simulink model "asbCubeSatACS"  (R2025b)
settings: Solver=FixedStepDiscrete  StartTime=0.0  StopTime=1000  FixedStep=CubeSatTimeStep  RelTol=1e-3  EnableMultiTasking=on
libraries: sharedtransform x2, aerolibsatdyn x1, aerolibutil x1
settings Model: DataDictionary=asbCubeSatModelData.sldd  ExtModeAutoUpdateStatusClock=off  Creator=The MathWorks, Inc.  LastModifiedBy=alokahn
settings SolverCC: AlgebraicLoopSolver=TrustRegion  MaxZcPerStep=1.0
settings DataIOCC: LimitDataPoints=on  SaveFormat=Array  SaveOutput=off  SignalLogging=off  DSMLogging=off  SaveTime=off  ReturnWorkspaceOutputs=off
settings OptimizationCC: DefaultParameterBehavior=Inlined  OptimizeBlockIOStorage=off  BufferReuse=off  GlobalBufferReuse=off  ExpressionFolding=off  ExpressionDepthLimit=2147483647.0  LocalBlockOutputs=off  InitFltsAndDblsToZero=on  LifeSpan=inf  OptimizeDataStoreBuffers=off  BusAssignmentInplaceUpdate=off
settings DebuggingCC: ArtificialAlgebraicLoopMsg=none  SolverPrmCheckMsg=warning  FcnCallInpInsideContextMsg=warning  UnconnectedInputMsg=warning  UnconnectedOutputMsg=warning  UnconnectedLineMsg=warning  StateNameClashWarn=warning  PregeneratedLibrarySubsystemCodeDiagnostic=none  SFUnexpectedBacktrackingDiag=warning  SFNoUnconditionalDefaultTransitionDiag=warning  SFExecutionAtInitializationDiag=none  ArithmeticOperatorsInVariantConditions=warning
settings HardwareCC: ProdBitPerPointer=32.0  ProdBitPerSizeT=32.0  ProdBitPerPtrDiffT=32.0  ProdLargestAtomicFloat=None  ProdIntDivRoundTo=Undefined  ProdEndianess=Unspecified  ProdWordSize=32.0  ProdHWDeviceType=32-bit Generic
settings ModelReferenceCC: EnableRefExpFcnMdlSchedulingChecks=on  PropagateSignalLabelsOutOfModel=off
settings SFSimCC: SimUseLocalCustomCode=off
settings RTWCC: RTWUseLocalCustomCode=off  GPUComputeCapability=3.5  DLArmComputeVersion=19.05
settings CodeAppCC: StateflowObjectComments=on
settings GRTTargetCC: TargetFcnLib=ansi_tfl_tmw.mat  TargetLangStandard=C89/C90 (ANSI)  CombineOutputUpdateFcns=off  GRTInterface=on
settings ConfigComp: CovMetricSettings=dw  CovSaveCumulativeToWorkspaceVar=on  CovSaveSingleToWorkspaceVar=on  CovExternalEMLEnable=off

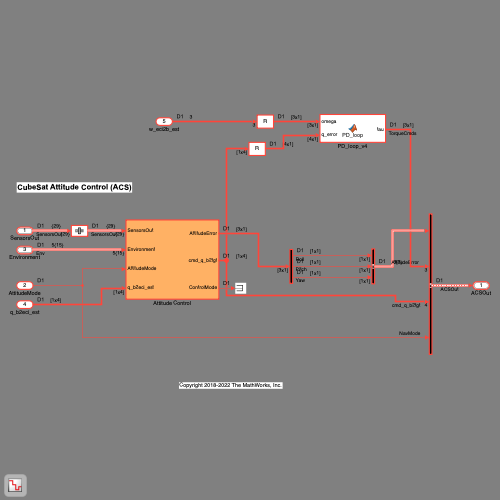
[thumbnail: Simulink's stored preview of the top-level diagram]
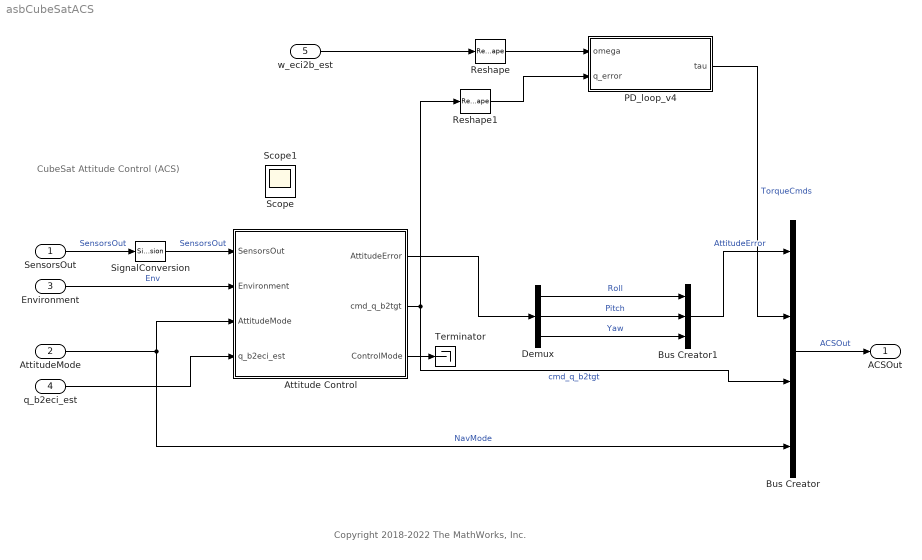
== system asbCubeSatACS ==
  note: Copyright 2018-2022 The MathWorks, Inc.
  note: CubeSat Attitude Control (ACS)
  SensorsOut : Inport  OutDataTypeStr=Bus: StatesOutBus
  AttitudeMode : Inport  Port=2  OutDataTypeStr=double  PortDimensions=1
  Environment : Inport  Port=3  OutDataTypeStr=Bus: EnvBus  PortDimensions=1
  q_b2eci_est : Inport  Port=4  PortDimensions=[1,4]  SampleTime=1
  w_eci2b_est : Inport  Port=5  SampleTime=1
  Attitude Control : Subsystem
  Bus Creator : BusCreator  Inputs=4  OutDataTypeStr=Bus: ACSOutBus  NonVirtualBus=on
  Bus Creator1 : BusCreator  Inputs=3  OutDataTypeStr=Bus: AttitudeErrorBus
  Demux : Demux  Outputs=3
  PD_loop_v4 : MATLAB Function  TreatAsAtomicUnit=on  SystemSampleTime=1
  Reshape : Reshape  OutputDimensionality=Customize  OutputDimensions=[3,1]
  Reshape1 : Reshape  OutputDimensionality=Customize  OutputDimensions=[4, 1]
  SignalConversion : SignalConversion  ConversionOutput=Virtual bus  OverrideOpt=off
  Terminator : Terminator
  ACSOut : Outport  OutDataTypeStr=Bus: ACSOutBus  PortDimensions=1  VectorParamsAs1DForOutWhenUnconnected=off  BusOutputAsStruct=on
  Scope : Scope
  Scope1 : Scope
      settings: ActiveDisplayYMinimum=-0.13646382044925889  ActiveDisplayYMaximum=3.23106670458966
  wires:
  Demux/1 -> Bus Creator1/1  "Roll"
  AttitudeMode/1 -> Bus Creator/4, Attitude Control/3("AttitudeMode ")  "NavMode"
  Demux/2 -> Bus Creator1/2  "Pitch"
  SensorsOut/1 -> SignalConversion/1  "SensorsOut"
  Bus Creator1/1 -> Bus Creator/1  "AttitudeError"
  Demux/3 -> Bus Creator1/3  "Yaw"
  Bus Creator/1 -> ACSOut/1  "ACSOut"
  Attitude Control/3(" ControlMode") -> Terminator/1
  Environment/1 -> Attitude Control/2(Environment)  "Env"
  Attitude Control/2(cmd_q_b2tgt) -> Reshape1/1, Bus Creator/3  "cmd_q_b2tgt"
  SignalConversion/1 -> Attitude Control/1("SensorsOut ")  "SensorsOut"
  Reshape/1 -> PD_loop_v4/1(omega)
  Attitude Control/1(AttitudeError) -> Demux/1
  PD_loop_v4/1(tau) -> Bus Creator/2  "TorqueCmds"
  Reshape1/1 -> PD_loop_v4/2(q_error)
  q_b2eci_est/1 -> Attitude Control/4(q_b2eci_est)
  w_eci2b_est/1 -> Reshape/1

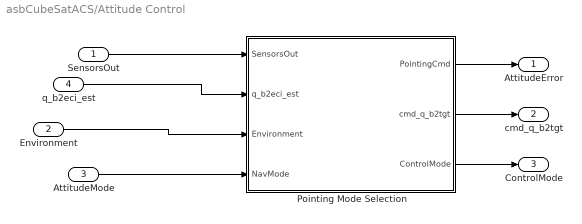
== system asbCubeSatACS/Attitude Control ==
  "SensorsOut " : Inport  OutDataTypeStr=Bus: StatesOutBus
  Environment : Inport  Port=2
  "AttitudeMode " : Inport  Port=3
  q_b2eci_est : Inport  Port=4  PortDimensions=[1,4]
  Pointing Mode Selection : Stateflow chart  RequirementInfo="{}  %GIDa_a065c7c8_537d_4123_b3cc_6e7e7008a32c"  TreatAsAtomicUnit=on
  AttitudeError : Outport  VectorParamsAs1DForOutWhenUnconnected=off
  cmd_q_b2tgt : Outport  Port=2  VectorParamsAs1DForOutWhenUnconnected=off
  " ControlMode" : Outport  Port=3  VectorParamsAs1DForOutWhenUnconnected=off
  wires:
  "SensorsOut "/1 -> Pointing Mode Selection/1(SensorsOut)
  Pointing Mode Selection/3(ControlMode) -> " ControlMode"/1
  "AttitudeMode "/1 -> Pointing Mode Selection/4(NavMode)
  Environment/1 -> Pointing Mode Selection/3(Environment)
  Pointing Mode Selection/1(PointingCmd) -> AttitudeError/1
  Pointing Mode Selection/2(cmd_q_b2tgt) -> cmd_q_b2tgt/1
  q_b2eci_est/1 -> Pointing Mode Selection/2(q_b2eci_est)

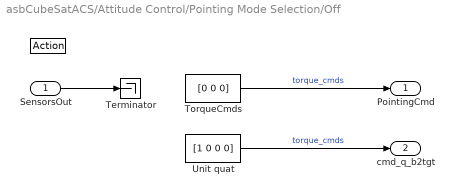
== system asbCubeSatACS/Attitude Control/Pointing Mode Selection/Off ==
  SensorsOut : Inport  OutDataTypeStr=Bus: StatesOutBus
  " " : ActionPort
      settings: CopyFcn=Stateflow.SLINSF.SimulinkMan.removeBlockPreDeleteFcn  PreDeleteFcn=Stateflow.SLINSF.SimulinkMan.unsafePredeleteFcn
  Terminator : Terminator
  TorqueCmds : Constant  Value=[0 0 0]
  Unit quat : Constant  Value=[1 0 0 0]
  PointingCmd : Outport  RequirementInfo="{}  %GIDa_4dc055f9_6cac_42e1_8ddb_4145586b89f5"  VectorParamsAs1DForOutWhenUnconnected=off
  cmd_q_b2tgt : Outport  RequirementInfo="{}  %GIDa_ca05d0a6_a581_4c3e_b3a0_cd281b586de8"  Port=2  VectorParamsAs1DForOutWhenUnconnected=off
  wires:
  SensorsOut/1 -> Terminator/1
  TorqueCmds/1 -> PointingCmd/1  "torque_cmds"
  Unit quat/1 -> cmd_q_b2tgt/1  "torque_cmds"

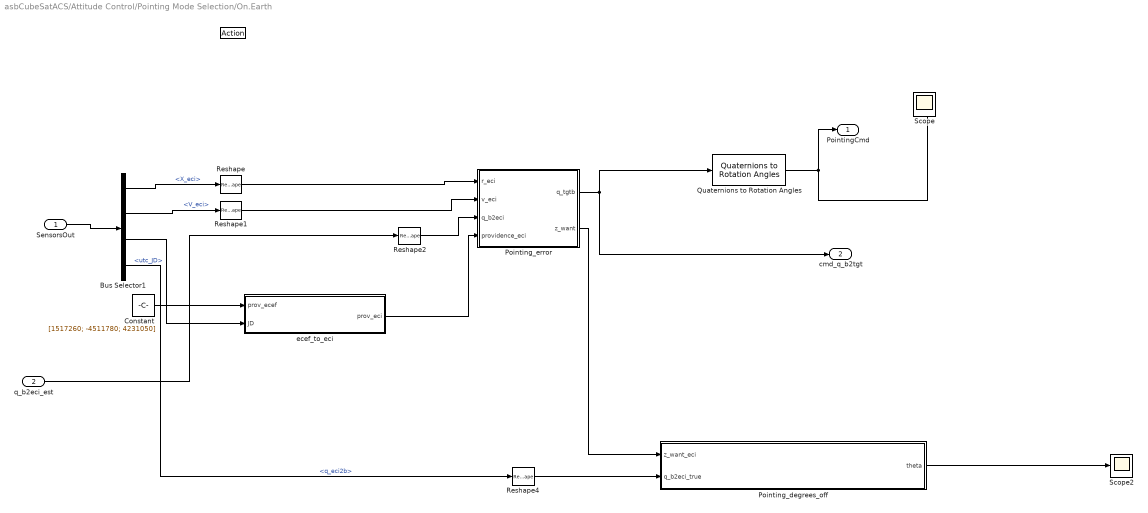
== system asbCubeSatACS/Attitude Control/Pointing Mode Selection/On.Earth ==
  SensorsOut : Inport  OutDataTypeStr=Bus: StatesOutBus
  q_b2eci_est : Inport  Port=2  PortDimensions=[1,4]
  " " : ActionPort
      settings: CopyFcn=Stateflow.SLINSF.SimulinkMan.removeBlockPreDeleteFcn  PreDeleteFcn=Stateflow.SLINSF.SimulinkMan.unsafePredeleteFcn
  Bus Selector1 : BusSelector  OutputSignals=X_eci,V_eci,utc_JD,q_eci2b
  Constant : Constant  Value=[1517260; -4511780; 4231050]
  Pointing_degrees_off : MATLAB Function  TreatAsAtomicUnit=on
  Pointing_error : MATLAB Function  TreatAsAtomicUnit=on
  Quaternions to Rotation Angles : sharedtransform/Quaternions to Rotation Angles  rotationOrder=XYZ  aMode=aMode
  Reshape : Reshape  OutputDimensionality=Column vector (2-D)
  Reshape1 : Reshape  OutputDimensionality=Column vector (2-D)
  Reshape2 : Reshape  OutputDimensionality=Customize  OutputDimensions=[1,4]
  Reshape4 : Reshape  OutputDimensionality=Customize  OutputDimensions=[1,4]
  Scope : Scope
      settings: ActiveDisplayYMinimum=-1.0198327701548264  ActiveDisplayYMaximum=2.2885054349185885  DataLoggingVariableName=ScopeData2
  Scope2 : Scope
      settings: ActiveDisplayYMinimum=-1.0711014685483513  ActiveDisplayYMaximum=15.846984806458  DataLoggingVariableName=ScopeData4
  ecef_to_eci : MATLAB Function  TreatAsAtomicUnit=on
  PointingCmd : Outport  VectorParamsAs1DForOutWhenUnconnected=off
  cmd_q_b2tgt : Outport  RequirementInfo="{}  %GIDa_69a01501_0b6a_41cf_b570_f5b49bb229cd"  Port=2  VectorParamsAs1DForOutWhenUnconnected=off
  wires:
  Quaternions to Rotation Angles/1 -> Scope/1, PointingCmd/1
  SensorsOut/1 -> Bus Selector1/1
  Bus Selector1/2 -> Reshape1/1  "<V_eci>"
  Bus Selector1/1 -> Reshape/1  "<X_eci>"
  q_b2eci_est/1 -> Reshape2/1
  Reshape/1 -> Pointing_error/1(r_eci)
  Reshape1/1 -> Pointing_error/2(v_eci)
  Reshape2/1 -> Pointing_error/3(q_b2eci)
  Pointing_error/1(q_tgtb) -> cmd_q_b2tgt/1, Quaternions to Rotation Angles/1
  Bus Selector1/3 -> ecef_to_eci/2(JD)  "<utc_JD>"
  Constant/1 -> ecef_to_eci/1(prov_ecef)
  ecef_to_eci/1(prov_eci) -> Pointing_error/4(providence_eci)
  Pointing_degrees_off/1(theta) -> Scope2/1
  Bus Selector1/4 -> Reshape4/1  "<q_eci2b>"
  Reshape4/1 -> Pointing_degrees_off/2(q_b2eci_true)
  Pointing_error/2(z_want) -> Pointing_degrees_off/1(z_want_eci)

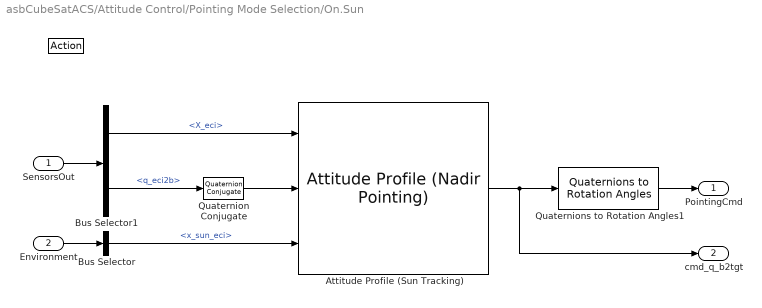
== system asbCubeSatACS/Attitude Control/Pointing Mode Selection/On.Sun ==
  SensorsOut : Inport  OutDataTypeStr=Bus: StatesOutBus
  Environment : Inport  Port=2  OutDataTypeStr=Bus: EnvBus
  " " : ActionPort
      settings: CopyFcn=Stateflow.SLINSF.SimulinkMan.removeBlockPreDeleteFcn  PreDeleteFcn=Stateflow.SLINSF.SimulinkMan.unsafePredeleteFcn
  Attitude Profile (Sun Tracking) : aerolibsatdyn/Attitude Profile (Nadir Pointing)  outputError=on  outputFinalAttitude=off  portFrame=ICRF  pointingMode=Custom  celestialTarget=Sun  tunablePointing=off  primaryAlignmentSrc=Dialog  primaryAlignment=[0 0 -1]  secondaryAlignmentSrc=Dialog  secondaryAlignment=[1 0 0]  constraintFrame=ICRF  primaryConstraintSrc=Port  primaryConstraint=[1 0 0]  secondaryConstraintSrc=Dialog  secondaryConstraint=[0 0 1]
  Bus Selector : BusSelector  OutputSignals=x_sun_eci
  Bus Selector1 : BusSelector  OutputSignals=X_eci,q_eci2b
  Quaternion Conjugate : aerolibutil/Quaternion Conjugate
  Quaternions to Rotation Angles1 : sharedtransform/Quaternions to Rotation Angles  rotationOrder=XYZ  aMode=aMode
  PointingCmd : Outport  VectorParamsAs1DForOutWhenUnconnected=off
  cmd_q_b2tgt : Outport  Port=2  VectorParamsAs1DForOutWhenUnconnected=off
  wires:
  Attitude Profile (Sun Tracking)/1 -> Quaternions to Rotation Angles1/1, cmd_q_b2tgt/1
  SensorsOut/1 -> Bus Selector1/1
  Environment/1 -> Bus Selector/1
  Quaternions to Rotation Angles1/1 -> PointingCmd/1
  Bus Selector/1 -> Attitude Profile (Sun Tracking)/3  "<x_sun_eci>"
  Quaternion Conjugate/1 -> Attitude Profile (Sun Tracking)/2
  Bus Selector1/2 -> Quaternion Conjugate/1  "<q_eci2b>"
  Bus Selector1/1 -> Attitude Profile (Sun Tracking)/1  "<X_eci>"

== matlab function asbCubeSatACS/Attitude Control/Pointing Mode Selection/On.Earth/Pointing_degrees_off ==
  data: z_want_eci input; theta output; q_b2eci_true input
function theta  = calc_error(z_want_eci, q_b2eci_true)
    R_body2eci_true = quat2rotm(q_b2eci_true);
    z_true_eci = R_body2eci_true(:, 3);

    z_true_eci = z_true_eci(:) / norm(z_true_eci);
    z_want_eci = z_want_eci / norm(z_want_eci);

    theta = rad2deg(acos(dot(z_true_eci, z_want_eci)));
end

== matlab function asbCubeSatACS/PD_loop_v4 ==
  data: omega input; q_error input; tau output
% INPUTS:
% omega - (3 x 1), deg/s: w_eci2b in body coordinates, that is angular velocity wr/ to eci
% written in body coordinates
% q_error - (4 x 1): error quaternion from pointing_error, scalar first

% RETURN:
% tau - torque in N-m, body coordinates


function tau = PD_loop(omega, q_error)

    arguments
        omega (3,1) double
        q_error (4, 1) double
    end
    %find shortest possible rotation
    if (q_error(1) < 0)
        q_error = -q_error;
    end

   
    angle = 2 * acos(q_error(1));

    if angle > 1e-12
        axis = q_error(2:4) / sin(angle/2);
    else
        axis = [0; 0; 0];
    end
    r_e = [axis; angle];
    % Convert 3x1 error omega vector back to axis-angle
    omega_rad = omega * (pi/180); % omega is in deg/s. converting to rad/s
    omega_mag = norm(omega_rad);
   
    if omega_mag > 1e-12
        omega_axis = omega_rad / omega_mag;
    else
        omega_axis = [0; 0; 0];
    end
    
    r_omega = [omega_axis; omega_mag];

    % PD controller
    Kp0 = 0.034;
    Kd0 = 0.42;
    max_tau = 5;
    min_tau = -5;
    I_body = [3.0054115e-02, -5.1674000e-05, 2.5075000e-05 ;-5.1674000e-05, 1.1430611e-02, -3.6481690e-03 ;2.5075000e-05, -3.6481690e-03, 2.3052295e-02];
    
    Kp = [Kp0, Kp0, Kp0];
    Kd = [Kd0, Kd0, Kd0];
    tau = zeros(3,1);

    for i = 1:3
        Pi = Kp(i) * r_e(4) * r_e(i);
        Di = Kd(i) * r_omega(4) * r_omega(i);
        tau(i) = Pi - Di;
    end
    tau = I_body * tau;
    tau = max(min(tau, max_tau), min_tau);
end

== matlab function asbCubeSatACS/Attitude Control/Pointing Mode Selection/On.Earth/ecef_to_eci ==
  data: prov_ecef input; prov_eci output; JD input
function prov_eci = eceftoeci(prov_ecef, JD)
    % Step 1: Unix time -> Julian Date

    % Step 2: Julian Date -> GMST (degrees)
    theta_deg = jd_to_gmst(JD);

    % Step 3: Build rotation matrix R_z(theta)
    theta = deg2rad(theta_deg);
    R = [ cos(theta), -sin(theta), 0; ...
          sin(theta),  cos(theta), 0; ...
          0,           0,          1];

    % Step 4: Rotate position
    prov_eci = R * prov_ecef;

end


% -------------------------------------------------------------------------
function theta_deg = jd_to_gmst(JD)
% JD_TO_GMST Compute Greenwich Mean Sidereal Time (degrees) from Julian Date.

    % Julian centuries since J2000.0
    T = (JD - 2451545.0) / 36525.0;

    % GMST in degrees
    theta_deg = 280.46061837 ...
              + 360.98564736629 * (JD - 2451545.0) ...
              + 0.000387933     * T^2 ...
              - T^3             / 38710000.0;

    % Reduce to [0, 360)
    theta_deg = mod(theta_deg, 360.0);
end

== stateflow chart asbCubeSatACS/Attitude Control/Pointing Mode Selection ==
  state On
    state Transition
    state Earth
    state Sun
    (default) -> Transition
    Transition -> Sun [order 2] : [NavMode == 2]
        | {ControlMode = 2;}
    Sun -> Transition : [NavMode == 1]
        | {ControlMode = 1;}
    Transition -> Earth [order 1] : [NavMode == 1]
        | {ControlMode = 2;}
    Earth -> Transition : [NavMode == 2]
        | {ControlMode = 1;}
  state Off
  (default) -> Off
  Off -> On : [NavMode ~= 0]
      | {ControlMode = 1;}
  On -> Off : [NavMode == 0]
      | {ControlMode = 0;}
  data: sf_internal_action_state_placeholder_data local double size=1 =0; sf_internal_action_state_placeholder_data local double size=1 =0; sf_internal_action_state_placeholder_data local double size=1 =0; SensorsOut input Bus: StatesOutBus; q_b2eci_est input; Environment input; NavMode input; PointingCmd output =[0 0 0]'; cmd_q_b2tgt output; ControlMode output

== matlab function asbCubeSatACS/Attitude Control/Pointing Mode Selection/On.Earth/Pointing_error ==
  data: r_eci input; q_tgtb output; v_eci input; q_b2eci input; providence_eci input; z_want output
% INPUTS:
% r_eci - (3 x 1): ECI coordinates of satellite position
% v_eci - (3 x 1): ECI velocity of satellite position
% q_b2eci - (1 x 4): quaternion of current orientation in body to eci,ACTIVE convention
% providence_eci - (1 x 3): ECI coordinates of Providence, Rhode Island
%
% RETURN:
% q_tgtb - (1 x 4): error quaternion, with axis in body coordinates
%
function [q_tgtb, z_want] = pointing_error(r_eci, v_eci, q_b2eci, providence_eci)
    persistent q_want_prev 
    if isempty(q_want_prev)
        q_want_prev = [1 0 0 0];   % initial guess, any unit quaternion
    end
    z_want = providence_eci - r_eci;
    z_want = z_want / norm(z_want);

    y_want = cross(z_want, v_eci);
    y_want = y_want / norm(y_want);

    x_want = cross(y_want, z_want);
    x_want = x_want / norm(x_want);

    R_want_eci = [x_want, y_want, z_want];

    q_want_eci = rotm2quat(R_want_eci);
    if dot(q_want_eci, q_want_prev) < 0
        q_want_eci = -q_want_eci;
    end
    q_want_prev = q_want_eci;   % store for next timestep
   
    q_tgtb = quatmultiply(quatinv(q_b2eci), q_want_eci);
  
end
